simulink model "sampleModel152"  (R2021b)
settings: Solver=VariableStepAuto  StartTime=0.0  StopTime=10.0  RelTol=1e-3
undefined symbols (not defined in the file or in its folder): DiscIntNeverNeededParam, Newton, Raphson
libraries: simulink x11, slpidlib x1
settings Model: Creator=user  LastModifiedBy=user

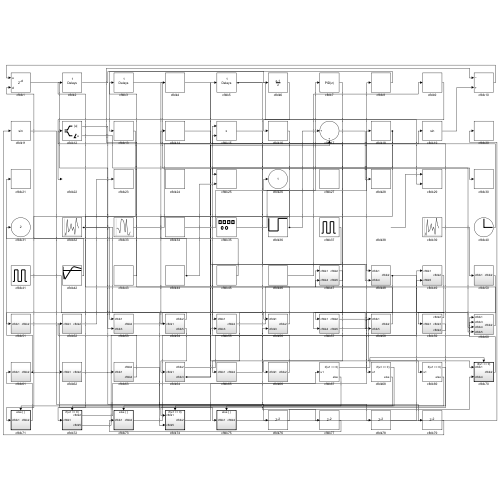
[thumbnail: Simulink's stored preview of the top-level diagram]
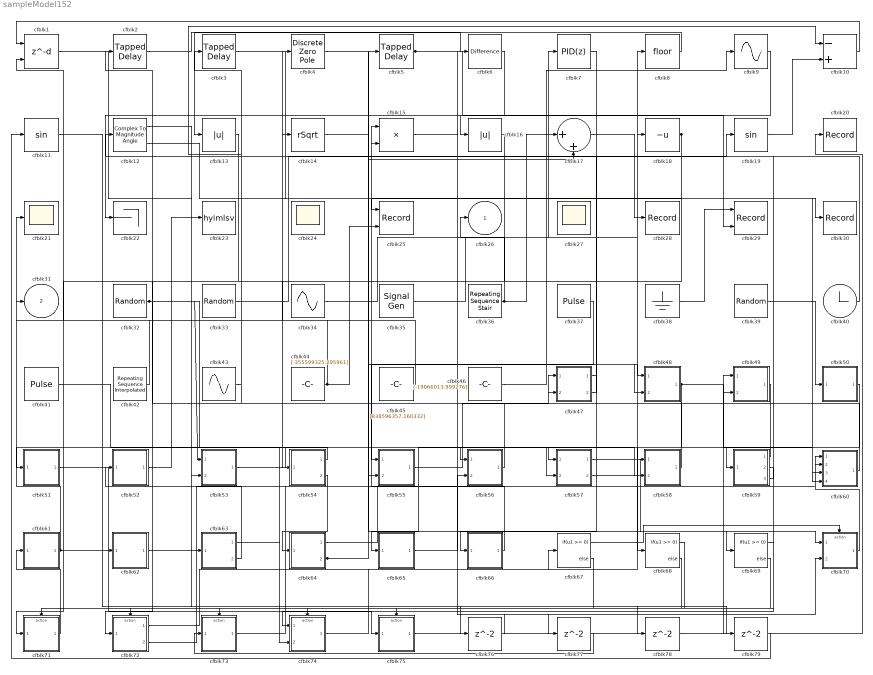
== system sampleModel152 ==
  cfblk1 : Delay  DelayLengthSource=Input port  SampleTime=1
      settings: InputPortMap=u0,p1
  cfblk10 : Sum  Inputs=-+
  cfblk11 : Trigonometry
  cfblk12 : ComplexToMagnitudeAngle
  cfblk13 : Abs
  cfblk14 : Sqrt  Operator=rSqrt  AlgorithmType=Newton-Raphson  SaturateOnIntegerOverflow=on
  cfblk15 : Product
  cfblk16 : Abs
  cfblk17 : Sum  Inputs=|++
  cfblk18 : UnaryMinus
  cfblk19 : Trigonometry
  cfblk2 : simulink/Discrete/Tapped Delay  vinit=0.0  samptime=-1  NumDelays=1  DelayOrder=Oldest  includeCurrent=off
  cfblk20 : Record  FileSettingsInternal="{\"entries\":[{\"content\":{\"excelSettings\":{\"content\":{},\"type\":\"Streamout.ExcelSettings\"}},\"type\":\"Streamout.FileSettingStorage\",\"uuid\":\"c47b721e-c502-495e-bc2c-23fa9a237a94\"}],\"packageUris\":[\"http://schema.mathworks.com/mf0/streamout_blocks/R2020a\"],\"version\":\"1.0\"}"  SignalsInternal="{\"entries\":[{\"content\":{\"signals\":[{\"content\":{\"blockPath\":[\"sampleModel152/cfblk20\"],\"channel\":[],\"dimensions\":[1],\"domain\":\"sampleModel152/cfblk20\",\"lineColor\":\"#d95319\",\"plots\":[1],\"port\":1,\"sid\":[\"\"],\"signalID\":5681,\"signalName\":\"cfblk75\"},\"type\":\"RecordBlkView.Signal\",\"uuid\":\"6b29897d-ef07-458a-9e41-9e53abe459e1\"}]},\"type\":\"RecordBlkView.InputSignals\",\"uuid\":\"85f72081-060a-407c-acbf-49079db1e742\"}],\"packageUris\":[\"http://schema.mathworks.com/mf0/streamout_blocks/R2020a\"],\"version\":\"1.0\"}"  VisualizationBindings="{\"sparklinesplugin\":{\"info\":[{\"bindingParametersList\":[],\"subplotID\":1}]}}"
  cfblk21 : Scope
  cfblk22 : Terminator
  cfblk23 : ToWorkspace  VariableName=hyimlsv  SaveFormat=Timeseries  SampleTime=-1
  cfblk24 : Scope
      settings: Floating=on
  cfblk25 : Record  FileSettingsInternal="{\"entries\":[{\"content\":{\"excelSettings\":{\"content\":{},\"type\":\"Streamout.ExcelSettings\"}},\"type\":\"Streamout.FileSettingStorage\",\"uuid\":\"8546e93f-715b-4185-8f36-8e6ff5d08789\"}],\"packageUris\":[\"http://schema.mathworks.com/mf0/streamout_blocks/R2020a\"],\"version\":\"1.0\"}"  Layout=[1 1]  SignalsInternal="{\"entries\":[{\"content\":{\"signals\":[{\"content\":{\"blockPath\":[\"sampleModel152/cfblk25\"],\"channel\":[],\"dimensions\":[1],\"domain\":\"sampleModel152/cfblk25\",\"lineColor\":\"#a2142f\",\"plots\":[1],\"port\":1,\"sid\":[\"\"],\"signalID\":5685,\"signalName\":\"cfblk18\"},\"type\":\"RecordBlkView.Signal\",\"uuid\":\"05ec31d6-fd38-4270-a47a-7922b4318d2e\"},{\"content\":{\"blockPath\":[\"sampleModel152/cfblk25\"],\"channel\":[],\"dimensions\":[1],\"domain\":\"sampleModel152/cfblk25\",\"lineColor\":\"#139fff\",\"plots\":[1],\"port\":2,\"sid\":[\"\"],\"signalID\":5689,\"signalName\":\"cfblk44\"},\"type\":\"RecordBlkView.Signal\",\"uuid\":\"24e062aa-9521-4ee9-b4ae-237d779aa3c6\"}]},\"type\":\"RecordBlkView.InputSignals\",\"uuid\":\"3a65de9b-1b80-4f85-81c6-176fcafaf8bb\"}],\"packageUris\":[\"http://schema.mathworks.com/mf0/streamout_blocks/R2020a\"],\"version\":\"1.0\"}"  VisualizationBindings="{\"xyplotplugin\":{\"info\":[{\"series\":[{\"bindingParametersList\":[{\"parameter\":\"X-Axis\",\"signalID\":5685,\"signalName\":\"cfblk18\"},{\"parameter\":\"Y-Axis\",\"signalID\":5689,\"signalName\":\"cfblk44\"}],\"seriesID\":2906}],\"subplotID\":1}]}}"  CompatibilityTag=XY
  cfblk27 : Scope
      settings: Floating=on
  cfblk28 : Record  FileSettingsInternal="{\"entries\":[{\"content\":{\"excelSettings\":{\"content\":{},\"type\":\"Streamout.ExcelSettings\"}},\"type\":\"Streamout.FileSettingStorage\",\"uuid\":\"6cacab10-1b5e-4cec-8765-deae7b2bdf96\"}],\"packageUris\":[\"http://schema.mathworks.com/mf0/streamout_blocks/R2020a\"],\"version\":\"1.0\"}"  SignalsInternal="{\"entries\":[{\"content\":{\"signals\":[{\"content\":{\"blockPath\":[\"sampleModel152/cfblk28\"],\"channel\":[],\"dimensions\":[1],\"domain\":\"sampleModel152/cfblk28\",\"lineColor\":\"#77ac30\",\"plots\":[1],\"port\":1,\"sid\":[\"\"],\"signalID\":5693,\"signalName\":\"cfblk17\"},\"type\":\"RecordBlkView.Signal\",\"uuid\":\"22faa192-de3f-4ae5-a89c-dffad7db9273\"}]},\"type\":\"RecordBlkView.InputSignals\",\"uuid\":\"bcc17e78-91b2-4c48-9e64-284fcdbe6e2b\"}],\"packageUris\":[\"http://schema.mathworks.com/mf0/streamout_blocks/R2020a\"],\"version\":\"1.0\"}"  VisualizationBindings="{\"sparklinesplugin\":{\"info\":[{\"bindingParametersList\":[],\"subplotID\":1}]}}"
  cfblk29 : Record  FileSettingsInternal="{\"entries\":[{\"content\":{\"excelSettings\":{\"content\":{},\"type\":\"Streamout.ExcelSettings\"}},\"type\":\"Streamout.FileSettingStorage\",\"uuid\":\"857bb119-ee54-4941-9ae6-14d668698a5d\"}],\"packageUris\":[\"http://schema.mathworks.com/mf0/streamout_blocks/R2020a\"],\"version\":\"1.0\"}"  Layout=[1 1]  SignalsInternal="{\"entries\":[{\"content\":{\"signals\":[{\"content\":{\"blockPath\":[\"sampleModel152/cfblk29\"],\"channel\":[],\"dimensions\":[1],\"domain\":\"sampleModel152/cfblk29\",\"lineColor\":\"#139fff\",\"plots\":[1],\"port\":2,\"sid\":[\"\"],\"signalID\":5697,\"signalName\":\"cfblk5\"},\"type\":\"RecordBlkView.Signal\",\"uuid\":\"1e2b0046-587d-4481-b4ab-f1abe963bb21\"},{\"content\":{\"blockPath\":[\"sampleModel152/cfblk29\"],\"channel\":[],\"dimensions\":[1],\"domain\":\"sampleModel152/cfblk29\",\"lineColor\":\"#a2142f\",\"plots\":[1],\"port\":1,\"sid\":[\"\"],\"signalID\":5705,\"signalName\":\"cfblk38\"},\"type\":\"RecordBlkView.Signal\",\"uuid\":\"379cc09d-3817-46e2-bf9c-e097dc89ccf1\"}]},\"type\":\"RecordBlkView.InputSignals\",\"uuid\":\"a85b44e6-0b77-4491-85d0-19c1b678a5df\"}],\"packageUris\":[\"http://schema.mathworks.com/mf0/streamout_blocks/R2020a\"],\"version\":\"1.0\"}"  VisualizationBindings="{\"xyplotplugin\":{\"info\":[{\"series\":[{\"bindingParametersList\":[{\"parameter\":\"X-Axis\",\"signalID\":5705,\"signalName\":\"cfblk38\"},{\"parameter\":\"Y-Axis\",\"signalID\":5697,\"signalName\":\"cfblk5\"}],\"seriesID\":9559}],\"subplotID\":1}]}}"  CompatibilityTag=XY
  cfblk3 : simulink/Discrete/Tapped Delay  vinit=0.0  samptime=-1  NumDelays=1  DelayOrder=Oldest  includeCurrent=off
  cfblk30 : Record  FileSettingsInternal="{\"entries\":[{\"content\":{\"excelSettings\":{\"content\":{},\"type\":\"Streamout.ExcelSettings\"}},\"type\":\"Streamout.FileSettingStorage\",\"uuid\":\"625a1501-f71e-49e9-9740-3205468b7647\"}],\"packageUris\":[\"http://schema.mathworks.com/mf0/streamout_blocks/R2020a\"],\"version\":\"1.0\"}"  SignalsInternal="{\"entries\":[{\"content\":{\"signals\":[{\"content\":{\"blockPath\":[\"sampleModel152/cfblk30\"],\"channel\":[],\"dimensions\":[1],\"domain\":\"sampleModel152/cfblk30\",\"lineColor\":\"#a2142f\",\"plots\":[1],\"port\":1,\"sid\":[\"\"],\"signalID\":5701,\"signalName\":\"cfblk3\"},\"type\":\"RecordBlkView.Signal\",\"uuid\":\"0052e0c4-d6db-45c4-b4ee-3624ae9909da\"}]},\"type\":\"RecordBlkView.InputSignals\",\"uuid\":\"7832ecd4-22f0-4a63-9437-63c94ca3da57\"}],\"packageUris\":[\"http://schema.mathworks.com/mf0/streamout_blocks/R2020a\"],\"version\":\"1.0\"}"  VisualizationBindings="{\"sparklinesplugin\":{\"info\":[{\"bindingParametersList\":[],\"subplotID\":1}]}}"
  cfblk32 : UniformRandomNumber  Minimum=[-5126869105.594875]  Maximum=[2308667735.973821]  Seed=[47372116.000000]  SampleTime=0.1
  cfblk33 : RandomNumber  Mean=[4779.321387]  Variance=[11400.363844]  Seed=[216975092.000000]  SampleTime=0.1
  cfblk34 : Sin  Amplitude=[343828945.107933]  Bias=[720499371.411561]  SampleTime=0
  cfblk35 : SignalGenerator  WaveForm=square  Amplitude=[-851904995.807157]
  cfblk36 : simulink/Sources/Repeating Sequence Stair  OutValues=[-92845703.845647, -13330513.068456]  tsamp=-1  OutMin=[]  OutMax=[]  OutDataTypeStr=double  OutputDataTypeScalingMode=double  OutDataType=fixdt(0,8)  ConRadixGroup=Best Precision: Vector-wise  OutScaling=2^-12
  cfblk37 : DiscretePulseGenerator  PulseType=Time based  Amplitude=[445116671.729583]  Period=[66463313.529924]  PulseWidth=5  PhaseDelay=[3.000000]
  cfblk38 : Ground
  cfblk39 : UniformRandomNumber  Minimum=[-1141066484.015148]  Maximum=[8379573596.915171]  Seed=[96492900.000000]  SampleTime=0.1
  cfblk4 : DiscreteZeroPole  Poles=[0 0.5]  Gain=1
  cfblk40 : Clock
  cfblk41 : DiscretePulseGenerator  PulseType=Time based  Amplitude=[-644647574.954051]  Period=[6532110.493789]  PulseWidth=5  PhaseDelay=[6.000000]
  cfblk42 : simulink/Sources/Repeating Sequence Interpolated  OutValues=[-129751815.707003, -868503524.698792, 314474600.968764, 414289989.315585, 219991178.733641]  TimeValues=[0 0.1 0.5 0.6 1].'  LookUpMeth=Use Input Below  tsamp=0.01  OutMin=[]  OutMax=[]  OutDataTypeStr=double  OutputDataTypeScalingMode=double  OutDataType=fixdt(0,8)  OutScaling=2^-10
  cfblk43 : Sin  Amplitude=[431734842.538580]  Bias=[-356012344.991995]  SampleTime=0
  cfblk44 : Constant  Value=[-355599325.295961]  SampleTime=1
  cfblk45 : Constant  Value=[838596357.160332]  SampleTime=1
  cfblk46 : Constant  Value=[-19066013.999276]  SampleTime=1
  cfblk47 : Subsystem
  cfblk48 : Subsystem
  cfblk49 : Subsystem
  cfblk5 : simulink/Discrete/Tapped Delay  vinit=0.0  samptime=-1  NumDelays=1  DelayOrder=Oldest  includeCurrent=off
  cfblk50 : Subsystem
  cfblk51 : Subsystem
  cfblk52 : Subsystem
  cfblk53 : Subsystem
  cfblk54 : Subsystem
  cfblk55 : Subsystem
  cfblk56 : Subsystem
  cfblk57 : Subsystem
  cfblk58 : Subsystem
  cfblk59 : Subsystem
  cfblk6 : simulink/Discrete/Difference  ICPrevInput=0.0  OutMin=[]  OutMax=[]  OutDataTypeStr=Inherit: Inherit via back propagation  OutDataType=fixdt(1, 16)  OutScaling=2^-10  DoSatur=off
  cfblk60 : Subsystem
  cfblk61 : Subsystem
  cfblk62 : Subsystem
  cfblk63 : Subsystem
  cfblk64 : Subsystem
  cfblk65 : Subsystem
  cfblk66 : Subsystem
  cfblk67 : If  IfExpression=u1 >= 0  SampleTime=1
  cfblk68 : If  IfExpression=u1 >= 0  SampleTime=1
  cfblk69 : If  IfExpression=u1 >= 0  SampleTime=1
  cfblk7 : slpidlib/PID Controller  Controller=PID  Form=Parallel  TimeDomain=Discrete-time  UseExternalTs=off  SampleTime=1  IntegratorMethod=Forward Euler  FilterMethod=Forward Euler  ControllerParametersSource=internal  P=1  I=1  D=0  UseFilter=on  N=100  TunerSelectOption=Transfer Function Based (PID Tuner App)  InitialConditionSource=internal  InitialConditionForIntegrator=0  InitialConditionForFilter=0  DifferentiatorICPrevScaledInput=0  ExternalReset=none  TrackingMode=off  Kt=1  LimitOutput=off  SatLimitsSource=internal  UpperSaturationLimit=inf  LowerSaturationLimit=-inf  LinearizeAsGain=off  AntiWindupMode=none  Kb=1  POutMin=[]  POutMax=[]  IOutMin=[]  IOutMax=[]  DOutMin=[]  DOutMax=[]  NOutMin=[]  NOutMax=[]  SumOutMin=[]  SumOutMax=[]  SaturationOutMin=[]  SaturationOutMax=[]  PParamMin=[]  PParamMax=[]  IParamMin=[]  IParamMax=[]  DParamMin=[]  DParamMax=[]  NParamMin=[]  NParamMax=[]  KbParamMin=[]  KbParamMax=[]  KtParamMin=[]  KtParamMax=[]  KbOutMin=[]  KbOutMax=[]  KtOutMin=[]  KtOutMax=[]  IntegratorOutMin=[]  IntegratorOutMax=[]  FilterOutMin=[]  FilterOutMax=[]  SumI1OutMin=[]  SumI1OutMax=[]  SumI2OutMin=[]  SumI2OutMax=[]  SumI3OutMin=[]  SumI3OutMax=[]  SumI4OutMin=[]  SumI4OutMax=[]  SumDOutMin=[]  SumDOutMax=[]  DifferentiatorOutMin=[]  DifferentiatorOutMax=[]  FilterDiffOutCoefMin=[]  FilterDiffOutCoefMax=[]  ReciprocalOutMin=[]  ReciprocalOutMax=[]  SumDenOutMin=[]  SumDenOutMax=[]  SumNumOutMin=[]  SumNumOutMax=[]  DivideOutMin=[]  DivideOutMax=[]  UdiffTsProdOutMin=[]  UdiffTsProdOutMax=[]  NTsProdOutMin=[]  NTsProdOutMax=[]  UintegralTsProdOutMin=[]  UintegralTsProdOutMax=[]  UngainTsProdOutMin=[]  UngainTsProdOutMax=[]  IntegratorContinuousStateAttributes=''  IntegratorStateMustResolveToSignalObject=off  IntegratorRTWStateStorageClass=Auto  FilterContinuousStateAttributes=''  FilterStateMustResolveToSignalObject=off  FilterRTWStateStorageClass=Auto  ParallelPVariant=InternalParameters  IdealPVariant=Disabled  IVariant=InternalParameters  DVariant=InternalParameters  IntegratorVariant=Discrete  SatVariant=Disabled  AWVariant=Passthrough  PCopyVariant=Disabled  TRVariant=Disabled  FdbkBlocksVariant=Forward  IdealPFdbkVariant=Disabled  SatFdbkVariant=Disabled  DerivativeFilterVariant=ForwardEulerFilter  NVariant=InternalParameters  NCopyVariant=Disabled  FilterICVariant=InternalICsFilter  IntegratorICVariant=InternalICs  ExternalResetVariant=Disabled  TRSumVariant=Passthrough  SumFdbkVariant=Disabled  SumVariant=Sum_PID  TsampFilterVariant=InternalTs  TsampNgainVariant=Passthrough  TsampIntegralVariant=Passthrough  ExternalSaturationOutDataTypeStr=Inherit: Same as second input
  cfblk70 : Subsystem  TreatAsAtomicUnit=on
  cfblk71 : Subsystem  TreatAsAtomicUnit=on
  cfblk72 : Subsystem  TreatAsAtomicUnit=on
  cfblk73 : Subsystem  TreatAsAtomicUnit=on
  cfblk74 : Subsystem  TreatAsAtomicUnit=on
  cfblk75 : Subsystem  TreatAsAtomicUnit=on
  cfblk{76..79} (4 alike) : Delay  SampleTime=1
  cfblk8 : Rounding
  cfblk9 : Sin  TimeSource=Use external signal  SampleTime=0
  cfblk26 : Outport
  cfblk31 : Outport  Port=2
  wires:
  cfblk72/1(cfblk2) -> cfblk8/1
  cfblk52/1(cfblk2) -> cfblk23/1
  cfblk8/1 -> cfblk13/1
  cfblk9/1 -> cfblk16/1
  cfblk43/1 -> cfblk10/1
  cfblk58/1(cfblk2) -> cfblk47/1(cfblk1)
  cfblk32/1 -> cfblk53/1(cfblk1), cfblk74/2(cfblk5)
  cfblk3/1 -> cfblk30/1
  cfblk33/1 -> cfblk19/1
  cfblk44/1 -> cfblk4/1, cfblk25/2
  cfblk42/1 -> cfblk21/1
  cfblk51/1(cfblk2) -> cfblk75/1(cfblk1)
  cfblk34/1 -> cfblk7/1
  cfblk74/1(cfblk2) -> cfblk67/1
  cfblk19/1 -> cfblk10/2
  cfblk46/1 -> cfblk9/1
  cfblk55/1(cfblk2) -> cfblk47/2(cfblk4)
  cfblk49/1(cfblk2) -> cfblk59/1(cfblk1)
  cfblk36/1 -> cfblk26/1, cfblk17/1
  cfblk6/1 -> cfblk22/1
  cfblk56/1(cfblk2) -> cfblk3/1
  cfblk71/1(cfblk2) -> cfblk61/1(cfblk1)
  cfblk35/1 -> cfblk18/1
  cfblk66/1(cfblk2) -> cfblk15/1
  cfblk38/1 -> cfblk29/1
  cfblk7/1 -> cfblk57/1(cfblk1)
  cfblk57/1(cfblk2) -> cfblk69/1
  cfblk47/1(cfblk2) -> cfblk66/1(cfblk1)
  cfblk72/2(cfblk5) -> cfblk5/1
  cfblk11/1 -> cfblk62/1(cfblk1)
  cfblk10/1 -> cfblk1/1
  cfblk70/1(cfblk2) -> cfblk60/1(cfblk1)
  cfblk40/1 -> cfblk15/2
  cfblk5/1 -> cfblk29/2, cfblk77/1
  cfblk47/2(cfblk5) -> cfblk14/1
  cfblk45/1 -> cfblk1/2
  cfblk63/2(cfblk4) -> cfblk52/1(cfblk1)
  cfblk53/1(cfblk2) -> cfblk56/1(cfblk1)
  cfblk14/1 -> cfblk70/1(cfblk1)
  cfblk61/1(cfblk2) -> cfblk31/1, cfblk76/1
  cfblk75/1(cfblk2) -> cfblk20/1
  cfblk4/1 -> cfblk48/1(cfblk1)
  cfblk16/1 -> cfblk54/1(cfblk1)
  cfblk1/1 -> cfblk53/2(cfblk3)
  cfblk65/1(cfblk2) -> cfblk56/2(cfblk3)
  cfblk60/1(cfblk2) -> cfblk2/1
  cfblk48/1(cfblk2) -> cfblk68/1, cfblk60/4(cfblk5)
  cfblk2/1 -> cfblk6/1
  cfblk64/1(cfblk2) -> cfblk49/2(cfblk5)
  cfblk59/1(cfblk2) -> cfblk57/2(cfblk4)
  cfblk54/1(cfblk2) -> cfblk51/1(cfblk1)
  cfblk17/1 -> cfblk28/1
  cfblk13/1 -> cfblk71/1(cfblk1)
  cfblk37/1 -> cfblk55/1(cfblk1)
  cfblk50/1(cfblk2) -> cfblk65/1(cfblk1)
  cfblk18/1 -> cfblk25/1, cfblk72/1(cfblk1)
  cfblk64/2(cfblk3) -> cfblk55/2(cfblk3), cfblk17/2
  cfblk73/1(cfblk2) -> cfblk60/2(cfblk3)
  cfblk15/1 -> cfblk48/2(cfblk4)
  cfblk12/1 -> cfblk63/1(cfblk1)
  cfblk57/2(cfblk5) -> cfblk58/1(cfblk1)
  cfblk59/2(cfblk3) -> cfblk74/1(cfblk1)
  cfblk12/2 -> cfblk60/3(cfblk4)
  cfblk39/1 -> cfblk50/1(cfblk1)
  cfblk54/2(cfblk5) -> cfblk64/1(cfblk1)
  cfblk59/3(cfblk4) -> cfblk12/1
  cfblk41/1 -> cfblk58/2(cfblk5)
  cfblk67/1 -> cfblk70/Action
  cfblk67/2 -> cfblk71/Action
  cfblk68/1 -> cfblk72/Action
  cfblk68/2 -> cfblk73/Action
  cfblk69/1 -> cfblk74/Action
  cfblk69/2 -> cfblk75/Action
  cfblk76/1 -> cfblk70/2(cfblk4)
  cfblk77/1 -> cfblk73/1(cfblk1)
  cfblk63/1(cfblk2) -> cfblk78/1
  cfblk78/1 -> cfblk49/1(cfblk1)
  cfblk62/1(cfblk2) -> cfblk79/1
  cfblk79/1 -> cfblk11/1

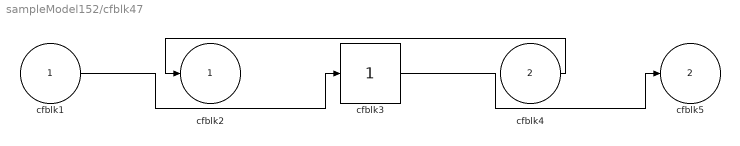
== system sampleModel152/cfblk47 ==
  cfblk1 : Inport
  cfblk4 : Inport  Port=2
  cfblk3 : simulink/Math Operations/Slider Gain  gain=1  low=0  high=2
  cfblk2 : Outport
  cfblk5 : Outport  Port=2
  wires:
  cfblk4/1 -> cfblk2/1
  cfblk3/1 -> cfblk5/1
  cfblk1/1 -> cfblk3/1

== system sampleModel152/cfblk48 ==
  cfblk1 : Inport
  cfblk4 : Inport  Port=2
  cfblk3 : DiscreteIntegrator  ICPrevOutput=DiscIntNeverNeededParam  ICPrevScaledInput=DiscIntNeverNeededParam
  cfblk2 : Outport
  wires:
  cfblk3/1 -> cfblk2/1
  cfblk4/1 -> cfblk3/1

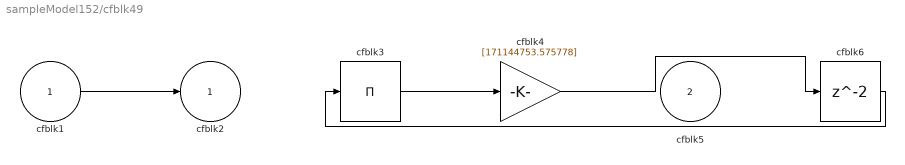
== system sampleModel152/cfblk49 ==
  cfblk1 : Inport
  cfblk5 : Inport  Port=2
  cfblk3 : Product  Inputs=*
  cfblk4 : Gain  Gain=[171144753.575778]
  cfblk6 : Delay  SampleTime=1
  cfblk2 : Outport
  wires:
  cfblk3/1 -> cfblk4/1
  cfblk1/1 -> cfblk2/1
  cfblk4/1 -> cfblk6/1
  cfblk6/1 -> cfblk3/1

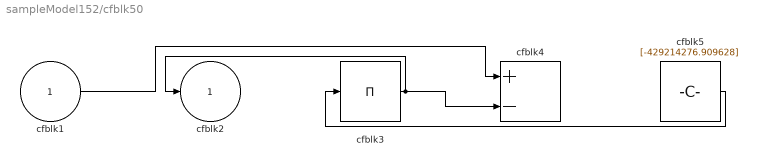
== system sampleModel152/cfblk50 ==
  cfblk1 : Inport
  cfblk3 : Product  Inputs=*
  cfblk4 : Sum  Inputs=+-
  cfblk5 : Constant  Value=[-429214276.909628]  SampleTime=1
  cfblk2 : Outport
  wires:
  cfblk3/1 -> cfblk2/1, cfblk4/2
  cfblk5/1 -> cfblk3/1
  cfblk1/1 -> cfblk4/1

== system sampleModel152/cfblk51 ==
  cfblk1 : Inport
  cfblk3 : Constant  Value=[610765290.185896]  SampleTime=1
  cfblk2 : Outport
  wires:
  cfblk3/1 -> cfblk2/1

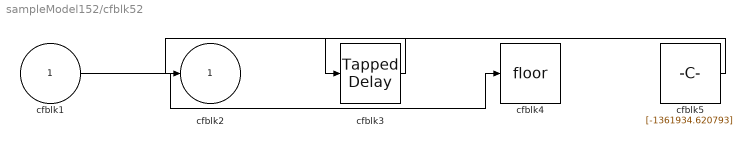
== system sampleModel152/cfblk52 ==
  cfblk1 : Inport
  cfblk3 : simulink/Discrete/Tapped Delay  vinit=0.0  samptime=-1  NumDelays=1  DelayOrder=Oldest  includeCurrent=off
  cfblk4 : Rounding
  cfblk5 : Constant  Value=[-1361934.620793]  SampleTime=1
  cfblk2 : Outport
  wires:
  cfblk5/1 -> cfblk3/1
  cfblk1/1 -> cfblk4/1
  cfblk3/1 -> cfblk2/1

== system sampleModel152/cfblk53 ==
  cfblk1 : Inport
  cfblk3 : Inport  Port=2
  cfblk2 : Outport
  wires:
  cfblk3/1 -> cfblk2/1

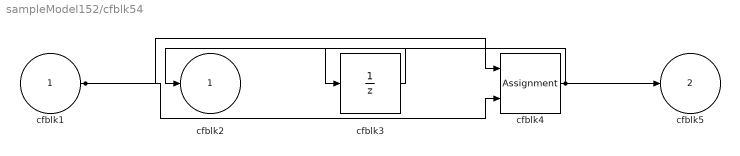
== system sampleModel152/cfblk54 ==
  cfblk1 : Inport
  cfblk3 : UnitDelay  HasFrameUpgradeWarning=on
  cfblk4 : Assignment  DiagnosticForDimensions=Warning  IndexOptions=Index vector (dialog)  Indices=1  OutputSizes=1
  cfblk2 : Outport
  cfblk5 : Outport  Port=2
  wires:
  cfblk3/1 -> cfblk2/1
  cfblk1/1 -> cfblk4/1, cfblk4/2
  cfblk4/1 -> cfblk5/1, cfblk3/1

== system sampleModel152/cfblk55 ==
  cfblk1 : Inport
  cfblk3 : Inport  Port=2
  cfblk2 : Outport
  wires:
  cfblk1/1 -> cfblk2/1

== system sampleModel152/cfblk56 ==
  cfblk1 : Inport
  cfblk3 : Inport  Port=2
  cfblk2 : Outport
  wires:
  cfblk3/1 -> cfblk2/1

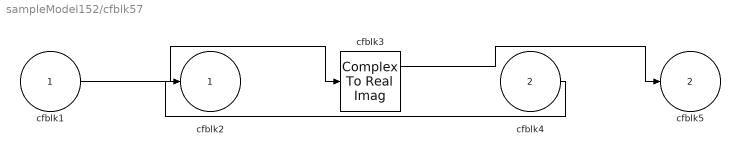
== system sampleModel152/cfblk57 ==
  cfblk1 : Inport
  cfblk4 : Inport  Port=2
  cfblk3 : ComplexToRealImag
  cfblk2 : Outport
  cfblk5 : Outport  Port=2
  wires:
  cfblk1/1 -> cfblk3/1
  cfblk4/1 -> cfblk2/1
  cfblk3/1 -> cfblk5/1

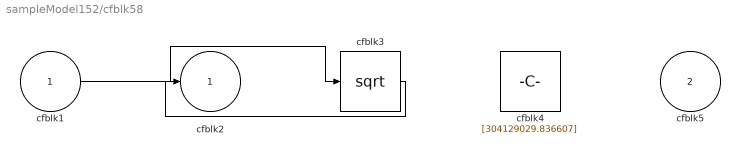
== system sampleModel152/cfblk58 ==
  cfblk1 : Inport
  cfblk5 : Inport  Port=2
  cfblk3 : Sqrt  SaturateOnIntegerOverflow=on
  cfblk4 : Constant  Value=[304129029.836607]  SampleTime=1
  cfblk2 : Outport
  wires:
  cfblk1/1 -> cfblk3/1
  cfblk3/1 -> cfblk2/1

== system sampleModel152/cfblk59 ==
  cfblk1 : Inport
  cfblk2 : Outport
  cfblk3 : Outport  Port=2
  cfblk4 : Outport  Port=3
  wires:
  cfblk1/1 -> cfblk3/1, cfblk4/1, cfblk2/1

== system sampleModel152/cfblk60 ==
  cfblk1 : Inport
  cfblk3 : Inport  Port=2
  cfblk4 : Inport  Port=3
  cfblk5 : Inport  Port=4
  cfblk2 : Outport
  wires:
  cfblk4/1 -> cfblk2/1

== system sampleModel152/cfblk61 ==
  cfblk1 : Inport
  cfblk3 : Math  Operator=hypot  SaturateOnIntegerOverflow=on
  cfblk2 : Outport
  wires:
  cfblk1/1 -> cfblk3/1, cfblk3/2
  cfblk3/1 -> cfblk2/1

== system sampleModel152/cfblk62 ==
  cfblk1 : Inport
  cfblk3 : simulink/Discrete/Transfer Fcn Real Zero  ZeroZ=0.75  ICPrevInput=0.0  DoSatur=off
      settings: SourceProductBaseCode=SL
  cfblk4 : Constant  Value=[749667734.627183]  SampleTime=1
  cfblk5 : Constant  Value=[-127191064.731779]  SampleTime=1
  cfblk2 : Outport
  wires:
  cfblk1/1 -> cfblk3/1
  cfblk5/1 -> cfblk2/1

== system sampleModel152/cfblk63 ==
  cfblk1 : Inport
  cfblk3 : Bias  Bias=[130101413.322657]
  cfblk2 : Outport
  cfblk4 : Outport  Port=2
  wires:
  cfblk1/1 -> cfblk2/1, cfblk3/1
  cfblk3/1 -> cfblk4/1

== system sampleModel152/cfblk64 ==
  cfblk1 : Inport
  cfblk2 : Outport
  cfblk3 : Outport  Port=2
  wires:
  cfblk1/1 -> cfblk3/1, cfblk2/1

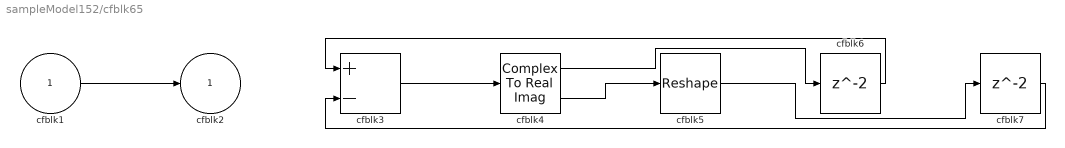
== system sampleModel152/cfblk65 ==
  cfblk1 : Inport
  cfblk3 : Sum  Inputs=+-
  cfblk4 : ComplexToRealImag
  cfblk5 : Reshape
  cfblk6 : Delay  SampleTime=1
  cfblk7 : Delay  SampleTime=1
  cfblk2 : Outport
  wires:
  cfblk4/2 -> cfblk5/1
  cfblk3/1 -> cfblk4/1
  cfblk1/1 -> cfblk2/1
  cfblk4/1 -> cfblk6/1
  cfblk6/1 -> cfblk3/1
  cfblk5/1 -> cfblk7/1
  cfblk7/1 -> cfblk3/2

== system sampleModel152/cfblk66 ==
  cfblk1 : Inport
  cfblk3 : Sum
  cfblk4 : Constant  Value=[-571991401.069180]  SampleTime=1
  cfblk2 : Outport
  wires:
  cfblk4/1 -> cfblk3/1
  cfblk1/1 -> cfblk2/1, cfblk3/2

== system sampleModel152/cfblk70 ==
  cfblk1 : Inport
  cfblk4 : Inport  Port=2
  Action Port : ActionPort  ActionPortLabel=if(u1 >= 0)
  cfblk3 : DiscreteFir
  cfblk2 : Outport
  wires:
  cfblk1/1 -> cfblk2/1
  cfblk4/1 -> cfblk3/1

== system sampleModel152/cfblk71 ==
  cfblk1 : Inport
  Action Port : ActionPort  ActionPortLabel=else
  cfblk3 : DiscreteFilter
  cfblk4 : ComplexToMagnitudeAngle
  cfblk2 : Outport
  wires:
  cfblk3/1 -> cfblk2/1
  cfblk4/1 -> cfblk3/1
  cfblk1/1 -> cfblk4/1

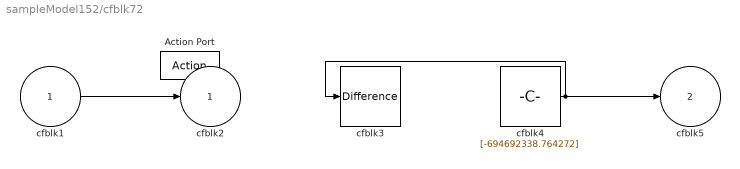
== system sampleModel152/cfblk72 ==
  cfblk1 : Inport
  Action Port : ActionPort  ActionPortLabel=if(u1 >= 0)
  cfblk3 : simulink/Discrete/Difference  ICPrevInput=0.0  OutMin=[]  OutMax=[]  OutDataTypeStr=Inherit: Inherit via back propagation  OutDataType=fixdt(1, 16)  OutScaling=2^-10  DoSatur=off
  cfblk4 : Constant  Value=[-694692338.764272]  SampleTime=1
  cfblk2 : Outport
  cfblk5 : Outport  Port=2
  wires:
  cfblk4/1 -> cfblk5/1, cfblk3/1
  cfblk1/1 -> cfblk2/1

== system sampleModel152/cfblk73 ==
  cfblk1 : Inport
  Action Port : ActionPort  ActionPortLabel=else
  cfblk3 : simulink/Discrete/Transfer Fcn Real Zero  ZeroZ=0.75  ICPrevInput=0.0  DoSatur=off
      settings: SourceProductBaseCode=SL
  cfblk2 : Outport
  wires:
  cfblk1/1 -> cfblk2/1, cfblk3/1

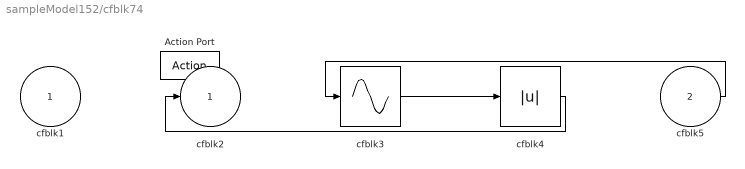
== system sampleModel152/cfblk74 ==
  cfblk1 : Inport
  cfblk5 : Inport  Port=2
  Action Port : ActionPort  ActionPortLabel=if(u1 >= 0)
  cfblk3 : Sin  TimeSource=Use external signal  SampleTime=0
  cfblk4 : Abs
  cfblk2 : Outport
  wires:
  cfblk5/1 -> cfblk3/1
  cfblk3/1 -> cfblk4/1
  cfblk4/1 -> cfblk2/1

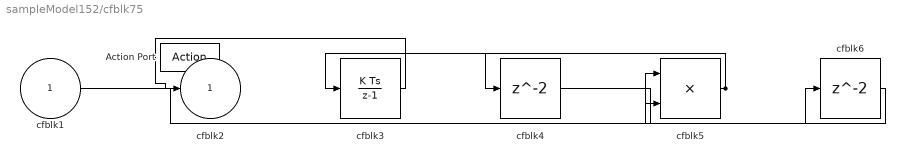
== system sampleModel152/cfblk75 ==
  cfblk1 : Inport
  Action Port : ActionPort  ActionPortLabel=else
  cfblk3 : DiscreteIntegrator  SampleTime=-1  ICPrevOutput=DiscIntNeverNeededParam  ICPrevScaledInput=DiscIntNeverNeededParam
  cfblk4 : Delay
  cfblk5 : Product  Inputs=**
  cfblk6 : Delay
  cfblk2 : Outport
  wires:
  cfblk5/1 -> cfblk4/1, cfblk3/1
  cfblk1/1 -> cfblk5/1
  cfblk3/1 -> cfblk2/1
  cfblk4/1 -> cfblk6/1
  cfblk6/1 -> cfblk5/2
